simulink model "MarsLander_2018a"  (R2018a)
settings: Solver=ode45  StartTime=0.0  StopTime=13  RelTol=1e-10  EnableMultiTasking=on
settings Model: Creator=liang  LastModifiedBy=bzhan
settings DataIOCC: LimitDataPoints=on  SaveFormat=Array  SignalLoggingSaveFormat=ModelDataLogs
settings OptimizationCC: ExpressionDepthLimit=2147483647  LifeSpan=inf
settings DebuggingCC: UnderspecifiedInitializationDetection=Classic  MergeDetectMultiDrivingBlocksExec=none  SolverPrmCheckMsg=warning  FcnCallInpInsideContextMsg=warning  StateNameClashWarn=warning  SFUnexpectedBacktrackingDiag=warning  SFNoUnconditionalDefaultTransitionDiag=warning  SFExecutionAtInitializationDiag=none
settings HardwareCC: ProdBitPerPointer=32  ProdBitPerSizeT=32  ProdBitPerPtrDiffT=32  ProdLargestAtomicFloat=None  ProdIntDivRoundTo=Undefined  ProdEndianess=Unspecified  ProdWordSize=32  ProdHWDeviceType=32-bit Generic
settings ModelReferenceCC: PropagateSignalLabelsOutOfModel=off
settings CodeAppCC: StateflowObjectComments=on
settings GRTTargetCC: TargetLangStandard=C89/C90 (ANSI)
settings ConfigComp: CovMetricSettings=dw  CovHtmlReporting=on  CovSaveCumulativeToWorkspaceVar=on  CovSaveSingleToWorkspaceVar=on  CovExternalEMLEnable=off

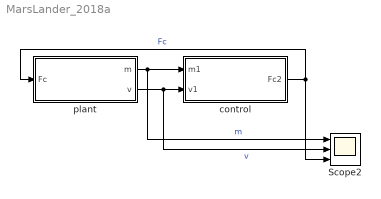
== system MarsLander_2018a ==
  Scope2 : Scope  NumInputPorts=3
  control : Subsystem
  plant : Subsystem
  wires:
  plant/1(m) -> Scope2/1, control/1(m1)  "m"
  plant/2(v) -> Scope2/2, control/2(v1)  "v"
  control/1(Fc2) -> plant/1(Fc), Scope2/3  "Fc"

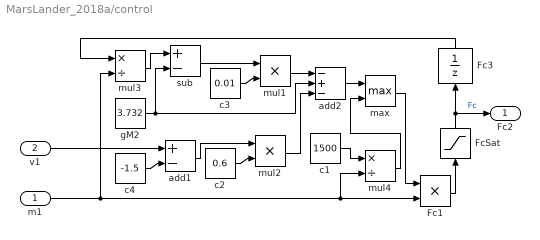
== system MarsLander_2018a/control ==
  m1 : Inport
  v1 : Inport  Port=2
  Fc1 : Product  Inputs=**  SampleTime=0.128
  Fc3 : UnitDelay  InitialCondition=2835  SampleTime=0.128  HasFrameUpgradeWarning=on
  FcSat : Saturate  UpperLimit=5000  LowerLimit=1500  SampleTime=0.128
  add1 : Sum  Inputs=+-  SampleTime=0.128
  add2 : Sum  Inputs=-+-  SampleTime=0.128
  c1 : Constant  Value=1500
  c2 : Constant  Value=0.6
  c3 : Constant  Value=0.01
  c4 : Constant  Value=-1.5
  gM2 : Constant  Value=3.732
  max : MinMax  Function=max  Inputs=2  SampleTime=0.128
  mul1 : Product  Inputs=**  SampleTime=0.128
  mul2 : Product  Inputs=**  SampleTime=0.128
  mul3 : Product  Inputs=*/  SampleTime=0.128
  mul4 : Product  Inputs=*/  SampleTime=0.128
  sub : Sum  Inputs=+-  SampleTime=0.128
  Fc2 : Outport
  wires:
  mul3/1 -> sub/1
  gM2/1 -> add2/2, sub/2
  sub/1 -> mul1/1
  c3/1 -> mul1/2
  c4/1 -> add1/2
  add1/1 -> mul2/1
  c2/1 -> mul2/2
  mul2/1 -> add2/3
  v1/1 -> add1/1
  add2/1 -> max/1
  Fc1/1 -> FcSat/1
  Fc3/1 -> mul3/1
  mul1/1 -> add2/1
  m1/1 -> mul3/2, Fc1/2, mul4/2
  FcSat/1 -> Fc3/1, Fc2/1  "Fc"
  max/1 -> Fc1/1
  c1/1 -> mul4/1
  mul4/1 -> max/2

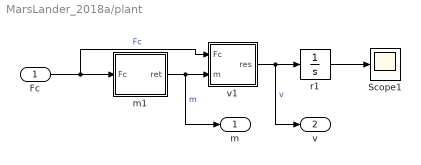
== system MarsLander_2018a/plant ==
  Fc : Inport
  Scope1 : Scope
  m1 : Subsystem
  r1 : Integrator  InitialCondition=20
  v1 : Subsystem
  m : Outport
  v : Outport  Port=2
  wires:
  m1/1(ret) -> v1/2(m), m/1  "m"
  v1/1(res) -> v/1, r1/1  "v"
  Fc/1 -> v1/1(Fc), m1/1(Fc)  "Fc"
  r1/1 -> Scope1/1

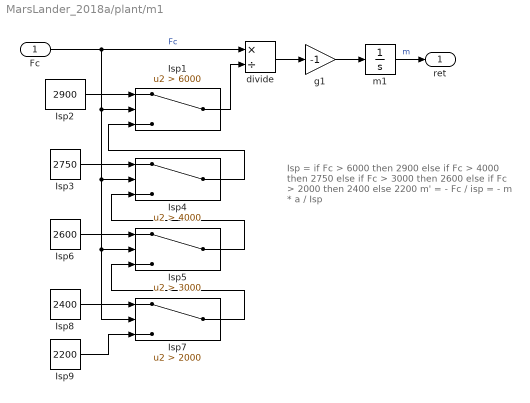
== system MarsLander_2018a/plant/m1 ==
  note: Isp = if Fc > 6000 then 2900 else
      | if Fc > 4000 then 2750 else
      | if Fc > 3000 then 2600 else
      | if Fc > 2000 then 2400 else 2200
      |
      | m' = - Fc / isp = - m * a / Isp
  Fc : Inport
  Isp1 : Switch  Criteria=u2 > Threshold  Threshold=6000  SampleTime=0
  Isp2 : Constant  Value=2900
  Isp3 : Constant  Value=2750
  Isp4 : Switch  Criteria=u2 > Threshold  Threshold=4000  SampleTime=0
  Isp5 : Switch  Criteria=u2 > Threshold  Threshold=3000  SampleTime=0
  Isp6 : Constant  Value=2600
  Isp7 : Switch  Criteria=u2 > Threshold  Threshold=2000  SampleTime=0
  Isp8 : Constant  Value=2400
  Isp9 : Constant  Value=2200
  divide : Product  Inputs=*/  SampleTime=0
  g1 : Gain  Gain=-1  SampleTime=0
  m1 : Integrator  InitialCondition=759.5
  ret : Outport
  wires:
  Fc/1 -> divide/1, Isp7/2, Isp5/2, Isp4/2, Isp1/2  "Fc"
  divide/1 -> g1/1
  g1/1 -> m1/1
  m1/1 -> ret/1  "m"
  Isp2/1 -> Isp1/1
  Isp1/1 -> divide/2
  Isp3/1 -> Isp4/1
  Isp4/1 -> Isp1/3
  Isp6/1 -> Isp5/1
  Isp5/1 -> Isp4/3
  Isp8/1 -> Isp7/1
  Isp7/1 -> Isp5/3
  Isp9/1 -> Isp7/3

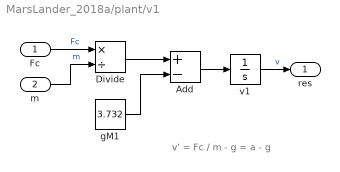
== system MarsLander_2018a/plant/v1 ==
  note: v' = Fc / m - g = a - g
  Fc : Inport
  m : Inport  Port=2
  Add : Sum  Inputs=+-  SampleTime=0
  Divide : Product  Inputs=*/  SampleTime=0
  gM1 : Constant  Value=3.732
  v1 : Integrator  InitialCondition=-1.5
  res : Outport
  wires:
  Fc/1 -> Divide/1  "Fc"
  m/1 -> Divide/2  "m"
  Divide/1 -> Add/1
  gM1/1 -> Add/2
  Add/1 -> v1/1
  v1/1 -> res/1  "v"
